simulink library "bcm"  (R2021b)
settings: Solver=VariableStepAuto  StartTime=0.0  StopTime=10.0  RelTol=1e-3
undefined symbols (not defined in the file): ENUM_ANTITHEFT_ALARM, ENUM_ANTITHEFT_ARM, ENUM_ANTITHEFT_DISARM, ENUM_ANTITHEFT_WAIT, ENUM_GEARPOSNTOCAN_P, ENUM_PDKEYRAWLULOCK_INUNLOCK, ENUM_PDKEYRAWPS_INPS, ENUM_POWERSTA_ON, ENUM_POWERSTA_READY, ENUM_POWERSTA_STANDBY, ENUM_PWRSTASW_ON, ENUM_PWRSTASW_READY, ENUM_SYSMODE_DEVELOPING, ENUM_SYSMODE_PRODUCT, ENUM_VEHICLETYPE_D21, ENUM_VEHICLETYPE_D31F25, ENUM_VEHICLETYPE_D31HAWD, ENUM_VEHICLETYPE_D31HRWD, ENUM_VEHICLETYPE_D31L24, FALSE, KBCM_ACCSwcPrsTmr_s, KBCM_ALMBrightnessDark_enum, KBCM_AmbBlue_enum, KBCM_AmbBreathT_ms, KBCM_AmbGreen_enum, KBCM_AmbMidPple_enum, KBCM_AmbRed_enum, KBCM_AmbTempCtrlEN_flg, KBCM_AmbTempT_s, KBCM_AmbWelModeENWait_s, KBCM_Antitheft_enum_ovrdflg, KBCM_Antitheft_enum_ovrdval, KBCM_APMDoorCtrlSta_flg_ovrdflg, KBCM_APMDoorCtrlSta_flg_ovrdval, KBCM_CmdKeepT_s, KBCM_CSWLightRstDebT_s, KBCM_CSWTurnLPRstT_s, KBCM_CycleTimeSet_s, KBCM_DelayTSW_flg, KBCM_DiagDRLOFF_flg, KBCM_DiagFLTC_mA, KBCM_DiagFMHT_s, KBCM_DiagFRTC_mA, KBCM_DiagRLTC_mA, KBCM_DiagRRTC_mA, KBCM_DrAPMRetryTimes_cnt, KBCM_DrOpenWdwOT_s, KBCM_DrOpenWdwReady_s, KBCM_DutyCycleSet_cnt, KBCM_DutyOverride_flg, KBCM_DutyOverride_val, KBCM_ESSOffT_ms, KBCM_ESSOnT_ms, KBCM_FDCDKCReDetectT_K, KBCM_FDCDKCUSSFilterT_K, KBCM_HandleLampKeepT_s, KBCM_IVIRstHoldT_ms, KBCM_IVIRstTriggerT_ms, KBCM_ONDelayT_ms, KBCM_RAPSAbnFlashOFFT_ms ... (+51)
libraries: simulink x402, $bdroot x10, hcu_lib x2
(part 11 of 14)

== system bcm/BCM/BCM/Personal_Setting/PTG/VALUE_TYPE_FlasherSignal ==
  UserNow : Inport
  Loadbar : Inport  Port=2
  iviCMD : Inport  Port=3
  EEP_Set12 : Inport  Port=4
  EEP_Set34 : Inport  Port=5
  EEP_Set57 : Inport  Port=6
  VINP_CANMsgValidIVI2_flg : Inport  Port=7
  NoReqV : Inport  Port=8
  Default : Inport  Port=9
  AND11 : Logic  Operator=OR  AllPortsSameDT=off  OutDataTypeStr=boolean
  Bitwise AND{1..4,11..12} (6 alike) : simulink/Logic and Bit Operations/Bitwise Operator  logicop=AND  UseBitMask=on  BitMask=bin2dec('11111111')  BitMaskRealWorld=Stored Integer
  Bitwise AND10 : simulink/Logic and Bit Operations/Bitwise Operator  logicop=AND  UseBitMask=on  BitMask=bin2dec('00111000')  BitMaskRealWorld=Stored Integer
  Bitwise AND5 : simulink/Logic and Bit Operations/Bitwise Operator  logicop=AND  UseBitMask=on  BitMask=bin2dec('00000111')  BitMaskRealWorld=Stored Integer
  Bitwise AND6 : simulink/Logic and Bit Operations/Bitwise Operator  logicop=AND  UseBitMask=on  BitMask=bin2dec('00111000')  BitMaskRealWorld=Stored Integer
  Bitwise AND7 : simulink/Logic and Bit Operations/Bitwise Operator  logicop=AND  UseBitMask=on  BitMask=bin2dec('00000111')  BitMaskRealWorld=Stored Integer
  Bitwise AND8 : simulink/Logic and Bit Operations/Bitwise Operator  logicop=AND  UseBitMask=on  BitMask=bin2dec('00000111')  BitMaskRealWorld=Stored Integer
  Bitwise AND9 : simulink/Logic and Bit Operations/Bitwise Operator  logicop=AND  UseBitMask=on  BitMask=bin2dec('00111000')  BitMaskRealWorld=Stored Integer
  Bitwise OR1 : simulink/Logic and Bit Operations/Bitwise Operator  logicop=OR  UseBitMask=off  NumInputPorts=2  BitMask=bin2dec('00000000000000000000')  BitMaskRealWorld=Stored Integer
  Bitwise OR2 : simulink/Logic and Bit Operations/Bitwise Operator  logicop=OR  UseBitMask=off  NumInputPorts=2  BitMask=bin2dec('00000000000000000000')  BitMaskRealWorld=Stored Integer
  Bitwise OR3 : simulink/Logic and Bit Operations/Bitwise Operator  logicop=OR  UseBitMask=off  NumInputPorts=2  BitMask=bin2dec('00000000000000000000')  BitMaskRealWorld=Stored Integer
  Compare To Constant5 : simulink/Logic and Bit Operations/Compare To Constant  relop===  const=0  OutDataTypeStr=boolean
  Constant : Constant  OutDataTypeStr=uint8
  Constant1 : Constant  Value=2  OutDataTypeStr=uint8
  Constant2 : Constant  Value=3  OutDataTypeStr=uint8
  Constant3 : Constant  Value=4  OutDataTypeStr=uint8
  Constant4 : Constant  Value=5  OutDataTypeStr=uint8
  Constant5 : Constant  Value=7  OutDataTypeStr=uint8
  Data Type Conversion{,1..14} (15 alike) : DataTypeConversion  OutDataTypeStr=uint8
  Detect Change1 : simulink/Logic and Bit Operations/Detect Change  vinit=0  OutDataTypeStr=boolean
  Detect Change7 : simulink/Logic and Bit Operations/Detect Change  vinit=0  OutDataTypeStr=boolean
  Logical Operator1 : Logic  Inputs=3  AllPortsSameDT=off  OutDataTypeStr=boolean
  Multiport Switch : MultiPortSwitch  Inputs=7  DataPortForDefault=Additional data port  DiagnosticForDefault=None
  NOT : Logic  Operator=NOT  AllPortsSameDT=off  OutDataTypeStr=boolean
  Relational Operator{,1..5} (6 alike) : RelationalOperator  Operator===  OutDataTypeStr=boolean  RndMeth=Simplest
  Relational Operator6 : RelationalOperator  Operator=<  OutDataTypeStr=boolean  RndMeth=Simplest
  Shift Arithmetic1 : ArithShift  BitShiftNumber=3  BitShiftDirection=Left
  Shift Arithmetic2 : ArithShift  BitShiftNumber=3  BitShiftDirection=Left
  Shift Arithmetic3 : ArithShift  BitShiftNumber=3  BitShiftDirection=Right
  Shift Arithmetic4 : ArithShift  BitShiftNumber=3  BitShiftDirection=Right
  Shift Arithmetic5 : ArithShift  BitShiftNumber=3  BitShiftDirection=Right
  Shift Arithmetic6 : ArithShift  BitShiftNumber=3  BitShiftDirection=Left
  Switch{,1..3,5,7..8,12..13} (9 alike) : Switch  Criteria=u2 ~= 0
  Switch{4,6,9..11} (5 alike) : Switch  Criteria=u2 > Threshold
  Unit Delay{1..13} (13 alike) : UnitDelay  SampleTime=-1  HasFrameUpgradeWarning=on
  Setting : Outport
  Set12 : Outport  Port=2
  Set34 : Outport  Port=3
  Set57 : Outport  Port=4
  wires:
  Default/1 -> Multiport Switch/7, Multiport Switch/9
  [Set7] -> Multiport Switch/8
  [Set5] -> Multiport Switch/6
  [Set4] -> Multiport Switch/5
  [Set3] -> Multiport Switch/4
  [Set2] -> Multiport Switch/3
  [Set1] -> Multiport Switch/2
  [Set] -> Switch2/1
  NOT/1 -> Switch1/2
  Switch8/1 -> [Set1], Unit Delay7/1
  Switch10/1 -> [Set5], Unit Delay4/1
  Switch7/1 -> Switch9/1
  Detect Change7/1 -> AND11/2
  Switch3/1 -> Switch4/1
  Relational Operator5/1 -> Unit Delay13/1
  Constant5/1 -> Relational Operator5/2
  [UserNow] -> Relational Operator5/1
  Relational Operator4/1 -> Unit Delay12/1
  Constant4/1 -> Relational Operator4/2
  [UserNow] -> Relational Operator4/1
  Relational Operator3/1 -> Unit Delay11/1
  Constant3/1 -> Relational Operator3/2
  [UserNow] -> Relational Operator3/1
  Relational Operator2/1 -> Unit Delay10/1
  Constant2/1 -> Relational Operator2/2
  [UserNow] -> Relational Operator2/1
  Relational Operator1/1 -> Unit Delay9/1
  Constant1/1 -> Relational Operator1/2
  [UserNow] -> Relational Operator1/1
  [Loadbar] -> Switch8/2
  Switch11/1 -> [Set7], Unit Delay5/1
  [Set] -> Switch7/1
  [Loadbar] -> Switch4/2
  Switch4/1 -> [Set2], Unit Delay2/1
  [UserNow] -> Relational Operator/1
  [Loadbar] -> Switch11/2
  [Loadbar] -> Switch6/2
  Constant/1 -> Relational Operator/2
  [Loadbar] -> Switch10/2
  [Set] -> Switch3/1
  [Set] -> Switch13/1
  Relational Operator/1 -> Unit Delay6/1
  [Set] -> Switch12/1
  [Loadbar] -> Switch9/2
  Switch9/1 -> [Set4], Unit Delay3/1
  [Set] -> Switch5/1
  Switch13/1 -> Switch10/1
  Switch5/1 -> Switch6/1
  Switch12/1 -> Switch11/1
  Switch2/1 -> Switch8/1
  Switch6/1 -> [Set3], Unit Delay8/1
  Relational Operator6/1 -> Logical Operator1/1
  Detect Change1/1 -> Logical Operator1/3
  iviCMD/1 -> Detect Change1/1, Relational Operator6/1, Switch/1
  Multiport Switch/1 -> Switch1/3
  Logical Operator1/1 -> Switch/2
  Switch1/1 -> Switch/3
  AND11/1 -> NOT/1
  Compare To Constant5/1 -> AND11/1
  UserNow/1 -> Multiport Switch/1, [UserNow], Detect Change7/1
  Loadbar/1 -> [Loadbar], Compare To Constant5/1
  Switch/1 -> Unit Delay1/1
  Unit Delay1/1 -> Switch1/1, [Set], Setting/1
  Unit Delay7/1 -> Switch2/3
  Unit Delay2/1 -> Switch3/3
  Unit Delay8/1 -> Switch5/3
  Unit Delay3/1 -> Switch7/3
  Unit Delay4/1 -> Switch13/3
  Unit Delay5/1 -> Switch12/3
  Unit Delay6/1 -> Switch2/2
  Unit Delay9/1 -> Switch3/2
  Unit Delay10/1 -> Switch5/2
  Unit Delay11/1 -> Switch7/2
  Unit Delay12/1 -> Switch13/2
  Unit Delay13/1 -> Switch12/2
  [EEP_Set1] -> Switch8/3
  [EEP_Set2] -> Switch4/3
  [EEP_Set3] -> Switch6/3
  [EEP_Set4] -> Switch9/3
  [EEP_Set5] -> Switch10/3
  [EEP_Set6] -> Switch11/3
  Bitwise AND1/1 -> Bitwise OR1/1
  Shift Arithmetic6/1 -> Bitwise AND2/1
  Data Type Conversion/1 -> Bitwise AND4/1
  Data Type Conversion3/1 -> Bitwise AND1/1
  Shift Arithmetic1/1 -> Bitwise AND11/1
  Data Type Conversion4/1 -> Shift Arithmetic1/1
  Bitwise AND2/1 -> Bitwise OR2/2
  Data Type Conversion1/1 -> Shift Arithmetic6/1
  Bitwise AND11/1 -> Bitwise OR1/2
  Bitwise AND4/1 -> Bitwise OR2/1
  Bitwise OR2/1 -> Set12/1
  Bitwise OR1/1 -> Set34/1
  [Set1] -> Data Type Conversion/1
  [Set2] -> Data Type Conversion1/1
  Bitwise AND9/1 -> Shift Arithmetic4/1
  Bitwise AND5/1 -> Data Type Conversion8/1
  Bitwise AND8/1 -> Data Type Conversion6/1
  Bitwise AND10/1 -> Shift Arithmetic5/1
  Bitwise AND7/1 -> Data Type Conversion10/1
  Shift Arithmetic5/1 -> Data Type Conversion11/1
  Shift Arithmetic4/1 -> Data Type Conversion7/1
  Bitwise AND6/1 -> Shift Arithmetic3/1
  Data Type Conversion6/1 -> [EEP_Set1]
  Data Type Conversion7/1 -> [EEP_Set2]
  Data Type Conversion8/1 -> [EEP_Set3]
  Data Type Conversion9/1 -> [EEP_Set4]
  Data Type Conversion10/1 -> [EEP_Set5]
  Data Type Conversion11/1 -> [EEP_Set6]
  EEP_Set34/1 -> Data Type Conversion13/1
  VINP_CANMsgValidIVI2_flg/1 -> Logical Operator1/2
  [Set3] -> Data Type Conversion3/1
  [Set4] -> Data Type Conversion4/1
  [Set7] -> Data Type Conversion5/1
  [Set5] -> Data Type Conversion2/1
  Bitwise OR3/1 -> Set57/1
  Bitwise AND12/1 -> Bitwise OR3/2
  Data Type Conversion5/1 -> Shift Arithmetic2/1
  Shift Arithmetic2/1 -> Bitwise AND12/1
  Data Type Conversion2/1 -> Bitwise AND3/1
  Bitwise AND3/1 -> Bitwise OR3/1
  EEP_Set57/1 -> Data Type Conversion14/1
  EEP_Set12/1 -> Data Type Conversion12/1
  Data Type Conversion12/1 -> Bitwise AND9/1, Bitwise AND8/1
  Data Type Conversion14/1 -> Bitwise AND10/1, Bitwise AND7/1
  Data Type Conversion13/1 -> Bitwise AND6/1, Bitwise AND5/1
  Shift Arithmetic3/1 -> Data Type Conversion9/1
  NoReqV/1 -> Relational Operator6/2

== system bcm/BCM/BCM/Personal_Setting/PTG/VALUE_TYPE_PTGUserSetMaxHeight ==
  UserNow : Inport
  Loadbar : Inport  Port=2
  VINP_PTGIsSetHeightSta_flg : Inport  Port=3
  VINP_PTGLeftHallPosn_cnt : Inport  Port=4
  EEP_Set1 : Inport  Port=5
  EEP_Set2 : Inport  Port=6
  EEP_Set3 : Inport  Port=7
  EEP_Set4 : Inport  Port=8
  EEP_Set5 : Inport  Port=9
  EEP_Set7 : Inport  Port=10
  NoReqV : Inport  Port=11
  Default : Inport  Port=12
  AND11 : Logic  Operator=OR  AllPortsSameDT=off  OutDataTypeStr=boolean
  Compare To Constant5 : simulink/Logic and Bit Operations/Compare To Constant  relop===  const=0  OutDataTypeStr=boolean
  Constant : Constant  OutDataTypeStr=uint8
  Constant1 : Constant  Value=2  OutDataTypeStr=uint8
  Constant2 : Constant  Value=3  OutDataTypeStr=uint8
  Constant3 : Constant  Value=4  OutDataTypeStr=uint8
  Constant4 : Constant  Value=5  OutDataTypeStr=uint8
  Constant5 : Constant  Value=7  OutDataTypeStr=uint8
  Detect Change7 : simulink/Logic and Bit Operations/Detect Change  vinit=0  OutDataTypeStr=boolean
  Detect Increase : simulink/Logic and Bit Operations/Detect Increase  vinit=0.0  OutDataTypeStr=boolean
  Logical Operator1 : Logic  AllPortsSameDT=off  OutDataTypeStr=boolean
  Multiport Switch : MultiPortSwitch  Inputs=7  DataPortForDefault=Additional data port  DiagnosticForDefault=None
  NOT : Logic  Operator=NOT  AllPortsSameDT=off  OutDataTypeStr=boolean
  Relational Operator{,1..5} (6 alike) : RelationalOperator  Operator===  OutDataTypeStr=boolean  RndMeth=Simplest
  Relational Operator6 : RelationalOperator  Operator=~=  OutDataTypeStr=boolean  RndMeth=Simplest
  Switch{,1..3,5,7..8,12..13} (9 alike) : Switch  Criteria=u2 ~= 0
  Switch{4,6,9..11} (5 alike) : Switch  Criteria=u2 > Threshold
  Unit Delay{1..13} (13 alike) : UnitDelay  SampleTime=-1  HasFrameUpgradeWarning=on
  Setting : Outport
  Set1 : Outport  Port=2
  Set2 : Outport  Port=3
  Set3 : Outport  Port=4
  Set4 : Outport  Port=5
  Set5 : Outport  Port=6
  Set7 : Outport  Port=7
  wires:
  VINP_PTGIsSetHeightSta_flg/1 -> Detect Increase/1
  Default/1 -> Multiport Switch/7, Multiport Switch/9
  [Set7] -> Multiport Switch/8
  [Set5] -> Multiport Switch/6
  [Set4] -> Multiport Switch/5
  [Set3] -> Multiport Switch/4
  [Set2] -> Multiport Switch/3
  [Set1] -> Multiport Switch/2
  [Set] -> Switch2/1
  NOT/1 -> Switch1/2
  Switch8/1 -> [Set1], Unit Delay7/1
  Switch10/1 -> [Set5], Unit Delay4/1
  Switch7/1 -> Switch9/1
  Detect Change7/1 -> AND11/2
  Switch3/1 -> Switch4/1
  Relational Operator5/1 -> Unit Delay13/1
  Constant5/1 -> Relational Operator5/2
  [UserNow] -> Relational Operator5/1
  Relational Operator4/1 -> Unit Delay12/1
  Constant4/1 -> Relational Operator4/2
  [UserNow] -> Relational Operator4/1
  Relational Operator3/1 -> Unit Delay11/1
  Constant3/1 -> Relational Operator3/2
  [UserNow] -> Relational Operator3/1
  Relational Operator2/1 -> Unit Delay10/1
  Constant2/1 -> Relational Operator2/2
  [UserNow] -> Relational Operator2/1
  Relational Operator1/1 -> Unit Delay9/1
  Constant1/1 -> Relational Operator1/2
  [UserNow] -> Relational Operator1/1
  [Loadbar] -> Switch8/2
  EEP_Set3/1 -> Switch6/3
  Switch11/1 -> [Set7], Unit Delay5/1
  EEP_Set4/1 -> Switch9/3
  [Set] -> Switch7/1
  [Loadbar] -> Switch4/2
  Switch4/1 -> [Set2], Unit Delay2/1
  [UserNow] -> Relational Operator/1
  EEP_Set2/1 -> Switch4/3
  EEP_Set5/1 -> Switch10/3
  [Loadbar] -> Switch11/2
  [Loadbar] -> Switch6/2
  Constant/1 -> Relational Operator/2
  [Loadbar] -> Switch10/2
  [Set] -> Switch3/1
  [Set] -> Switch13/1
  Relational Operator/1 -> Unit Delay6/1
  [Set] -> Switch12/1
  [Loadbar] -> Switch9/2
  EEP_Set7/1 -> Switch11/3
  Switch9/1 -> [Set4], Unit Delay3/1
  EEP_Set1/1 -> Switch8/3
  [Set] -> Switch5/1
  Switch13/1 -> Switch10/1
  Switch5/1 -> Switch6/1
  Switch12/1 -> Switch11/1
  Switch2/1 -> Switch8/1
  Switch6/1 -> [Set3], Unit Delay8/1
  NoReqV/1 -> Relational Operator6/1
  Relational Operator6/1 -> Logical Operator1/1
  Detect Increase/1 -> Logical Operator1/2
  VINP_PTGLeftHallPosn_cnt/1 -> Relational Operator6/2, Switch/1
  Multiport Switch/1 -> Switch1/3
  Logical Operator1/1 -> Switch/2
  Switch1/1 -> Switch/3
  [Set1] -> Set1/1
  [Set2] -> Set2/1
  [Set3] -> Set3/1
  [Set4] -> Set4/1
  [Set5] -> Set5/1
  [Set7] -> Set7/1
  AND11/1 -> NOT/1
  Compare To Constant5/1 -> AND11/1
  UserNow/1 -> Multiport Switch/1, [UserNow], Detect Change7/1
  Loadbar/1 -> [Loadbar], Compare To Constant5/1
  Switch/1 -> Unit Delay1/1
  Unit Delay1/1 -> Switch1/1, [Set], Setting/1
  Unit Delay7/1 -> Switch2/3
  Unit Delay2/1 -> Switch3/3
  Unit Delay8/1 -> Switch5/3
  Unit Delay3/1 -> Switch7/3
  Unit Delay4/1 -> Switch13/3
  Unit Delay5/1 -> Switch12/3
  Unit Delay6/1 -> Switch2/2
  Unit Delay9/1 -> Switch3/2
  Unit Delay10/1 -> Switch5/2
  Unit Delay11/1 -> Switch7/2
  Unit Delay12/1 -> Switch13/2
  Unit Delay13/1 -> Switch12/2

== system bcm/BCM/BCM/Personal_Setting/RoomLamp/TOGGLE_TYPE_RoomLampMode ==
  UserNow : Inport
  Loadbar : Inport  Port=2
  iviCMD : Inport  Port=3
  EEP_Set : Inport  Port=4
  Default : Inport  Port=5
  AND : Logic  AllPortsSameDT=off  OutDataTypeStr=boolean
  AND11 : Logic  Operator=OR  AllPortsSameDT=off  OutDataTypeStr=boolean
  Bitwise AND{,1..4} (5 alike) : simulink/Logic and Bit Operations/Bitwise Operator  logicop=AND  UseBitMask=on  BitMask=bin2dec('11111111')  BitMaskRealWorld=Stored Integer
  Bitwise AND10 : simulink/Logic and Bit Operations/Bitwise Operator  logicop=AND  UseBitMask=on  BitMask=bin2dec('00100000')  BitMaskRealWorld=Stored Integer
  Bitwise AND5 : simulink/Logic and Bit Operations/Bitwise Operator  logicop=AND  UseBitMask=on  BitMask=bin2dec('00000001')  BitMaskRealWorld=Stored Integer
  Bitwise AND6 : simulink/Logic and Bit Operations/Bitwise Operator  logicop=AND  UseBitMask=on  BitMask=bin2dec('00000010')  BitMaskRealWorld=Stored Integer
  Bitwise AND7 : simulink/Logic and Bit Operations/Bitwise Operator  logicop=AND  UseBitMask=on  BitMask=bin2dec('00000100')  BitMaskRealWorld=Stored Integer
  Bitwise AND8 : simulink/Logic and Bit Operations/Bitwise Operator  logicop=AND  UseBitMask=on  BitMask=bin2dec('00001000')  BitMaskRealWorld=Stored Integer
  Bitwise AND9 : simulink/Logic and Bit Operations/Bitwise Operator  logicop=AND  UseBitMask=on  BitMask=bin2dec('00010000')  BitMaskRealWorld=Stored Integer
  Bitwise OR2 : simulink/Logic and Bit Operations/Bitwise Operator  logicop=OR  UseBitMask=off  NumInputPorts=6  BitMask=bin2dec('00000000000000000000')  BitMaskRealWorld=Stored Integer
  Compare To Constant5 : simulink/Logic and Bit Operations/Compare To Constant  relop===  const=0  OutDataTypeStr=boolean
  Constant : Constant  OutDataTypeStr=uint8
  Constant1 : Constant  Value=2  OutDataTypeStr=uint8
  Constant2 : Constant  Value=3  OutDataTypeStr=uint8
  Constant3 : Constant  Value=4  OutDataTypeStr=uint8
  Constant4 : Constant  Value=5  OutDataTypeStr=uint8
  Constant5 : Constant  Value=7  OutDataTypeStr=uint8
  Data Type Conversion{,1..5} (6 alike) : DataTypeConversion  OutDataTypeStr=uint8
  Data Type Conversion{6..11} (6 alike) : DataTypeConversion  OutDataTypeStr=boolean
  Detect Change1 : simulink/Logic and Bit Operations/Detect Change  vinit=0  OutDataTypeStr=boolean
  Detect Increase : simulink/Logic and Bit Operations/Detect Increase  vinit=0.0  OutDataTypeStr=boolean
  Multiport Switch : MultiPortSwitch  Inputs=7  DataPortForDefault=Additional data port  DiagnosticForDefault=None
  NOT : Logic  Operator=NOT  IconShape=distinctive  AllPortsSameDT=off  OutDataTypeStr=boolean
  NOT1 : Logic  Operator=NOT  IconShape=distinctive  AllPortsSameDT=off  OutDataTypeStr=boolean
  Relational Operator{,1..5} (6 alike) : RelationalOperator  Operator===  OutDataTypeStr=boolean  RndMeth=Simplest
  Shift Arithmetic1 : ArithShift  BitShiftNumber=4  BitShiftDirection=Left
  Shift Arithmetic10 : ArithShift  BitShiftNumber=5  BitShiftDirection=Right
  Shift Arithmetic2 : ArithShift  BitShiftNumber=5  BitShiftDirection=Left
  Shift Arithmetic3 : ArithShift  BitShiftNumber=1  BitShiftDirection=Right
  Shift Arithmetic4 : ArithShift  BitShiftNumber=2  BitShiftDirection=Right
  Shift Arithmetic5 : ArithShift  BitShiftNumber=3  BitShiftDirection=Right
  Shift Arithmetic6 : ArithShift  BitShiftNumber=1  BitShiftDirection=Left
  Shift Arithmetic7 : ArithShift  BitShiftNumber=2  BitShiftDirection=Left
  Shift Arithmetic8 : ArithShift  BitShiftNumber=3  BitShiftDirection=Left
  Shift Arithmetic9 : ArithShift  BitShiftNumber=4  BitShiftDirection=Right
  Switch{,1..3,5,7,12..13} (8 alike) : Switch  Criteria=u2 ~= 0
  Switch{4,6,8..11} (6 alike) : Switch  Criteria=u2 > Threshold
  Unit Delay{1..4,6..14} (13 alike) : UnitDelay  SampleTime=-1  HasFrameUpgradeWarning=on
  Setting : Outport
  Set : Outport  Port=2
  wires:
  Default/1 -> Multiport Switch/7, Multiport Switch/9
  [Set7] -> Multiport Switch/8
  [Set5] -> Multiport Switch/6
  [Set4] -> Multiport Switch/5
  [Set3] -> Multiport Switch/4
  [Set2] -> Multiport Switch/3
  [Set1] -> Multiport Switch/2
  NOT1/1 -> Switch1/2
  Switch13/1 -> Switch10/1
  Multiport Switch/1 -> Switch1/3
  Loadbar/1 -> [Loadbar], Compare To Constant5/1
  Switch1/1 -> Switch/3
  UserNow/1 -> Multiport Switch/1, [UserNow], Detect Change1/1
  NOT/1 -> Switch/1
  iviCMD/1 -> Detect Increase/1
  [Set] -> Switch13/1
  [Loadbar] -> Switch4/2
  [Set] -> Switch12/1
  [UserNow] -> Relational Operator5/1
  Constant5/1 -> Relational Operator5/2
  [UserNow] -> Relational Operator/1
  [UserNow] -> Relational Operator1/1
  [Loadbar] -> Switch10/2
  Constant2/1 -> Relational Operator2/2
  [Loadbar] -> Switch11/2
  [Set] -> Switch3/1
  Constant/1 -> Relational Operator/2
  [Loadbar] -> Switch9/2
  [UserNow] -> Relational Operator2/1
  [UserNow] -> Relational Operator3/1
  Constant3/1 -> Relational Operator3/2
  [Set] -> Switch2/1
  [UserNow] -> Relational Operator4/1
  Constant1/1 -> Relational Operator1/2
  [Set] -> Switch7/1
  [Loadbar] -> Switch6/2
  [Set] -> Switch5/1
  [Loadbar] -> Switch8/2
  Constant4/1 -> Relational Operator4/2
  Compare To Constant5/1 -> AND11/1
  AND11/1 -> NOT1/1
  Switch/1 -> Unit Delay7/1
  Switch8/1 -> [Set1], Unit Delay6/1
  Switch2/1 -> Switch8/1
  Switch3/1 -> Switch4/1
  Switch4/1 -> [Set2], Unit Delay1/1
  Switch6/1 -> [Set3], Unit Delay11/1
  Switch5/1 -> Switch6/1
  Switch7/1 -> Switch9/1
  Switch9/1 -> [Set4], Unit Delay12/1
  Switch10/1 -> [Set5], Unit Delay13/1
  Switch12/1 -> Switch11/1
  Switch11/1 -> [Set7], Unit Delay14/1
  Unit Delay7/1 -> Setting/1, NOT/1, [Set], Switch1/1
  Relational Operator2/1 -> Unit Delay10/1
  Relational Operator3/1 -> Unit Delay2/1
  Relational Operator4/1 -> Unit Delay3/1
  Relational Operator5/1 -> Unit Delay4/1
  Data Type Conversion2/1 -> Shift Arithmetic7/1
  Data Type Conversion5/1 -> Shift Arithmetic2/1
  [Set4] -> Data Type Conversion3/1
  Shift Arithmetic8/1 -> Bitwise AND/1
  Shift Arithmetic2/1 -> Bitwise AND4/1
  Bitwise AND3/1 -> Bitwise OR2/5
  Bitwise AND1/1 -> Bitwise OR2/3
  Bitwise AND2/1 -> Bitwise OR2/2
  Shift Arithmetic6/1 -> Bitwise AND2/1
  Data Type Conversion4/1 -> Shift Arithmetic1/1
  Shift Arithmetic7/1 -> Bitwise AND1/1
  Shift Arithmetic1/1 -> Bitwise AND3/1
  [Set7] -> Data Type Conversion5/1
  Data Type Conversion/1 -> Bitwise OR2/1
  [Set2] -> Data Type Conversion1/1
  Data Type Conversion3/1 -> Shift Arithmetic8/1
  [Set1] -> Data Type Conversion/1
  [Set5] -> Data Type Conversion4/1
  Bitwise AND/1 -> Bitwise OR2/4
  Data Type Conversion1/1 -> Shift Arithmetic6/1
  Bitwise AND4/1 -> Bitwise OR2/6
  [Set3] -> Data Type Conversion2/1
  Bitwise OR2/1 -> Set/1
  Bitwise AND8/1 -> Shift Arithmetic5/1
  Bitwise AND6/1 -> Shift Arithmetic3/1
  Bitwise AND9/1 -> Shift Arithmetic9/1
  Bitwise AND10/1 -> Shift Arithmetic10/1
  Shift Arithmetic4/1 -> Data Type Conversion8/1
  Shift Arithmetic10/1 -> Data Type Conversion11/1
  Bitwise AND5/1 -> Data Type Conversion6/1
  Shift Arithmetic3/1 -> Data Type Conversion7/1
  Bitwise AND7/1 -> Shift Arithmetic4/1
  Shift Arithmetic9/1 -> Data Type Conversion10/1
  Shift Arithmetic5/1 -> Data Type Conversion9/1
  EEP_Set/1 -> [EEP_Set]
  [EEP_Set] -> Bitwise AND5/1
  [EEP_Set] -> Bitwise AND6/1
  [EEP_Set] -> Bitwise AND7/1
  [EEP_Set] -> Bitwise AND8/1
  [EEP_Set] -> Bitwise AND9/1
  [EEP_Set] -> Bitwise AND10/1
  Data Type Conversion6/1 -> [EEP_Set1]
  Data Type Conversion7/1 -> [EEP_Set2]
  Data Type Conversion8/1 -> [EEP_Set3]
  Data Type Conversion9/1 -> [EEP_Set4]
  Data Type Conversion10/1 -> [EEP_Set5]
  Data Type Conversion11/1 -> [EEP_Set6]
  [EEP_Set1] -> Switch8/3
  [EEP_Set2] -> Switch4/3
  [EEP_Set3] -> Switch6/3
  [EEP_Set4] -> Switch9/3
  [EEP_Set5] -> Switch10/3
  [EEP_Set6] -> Switch11/3
  Relational Operator/1 -> Unit Delay8/1
  Relational Operator1/1 -> Unit Delay9/1
  Unit Delay6/1 -> Switch2/3
  Unit Delay1/1 -> Switch3/3
  Unit Delay8/1 -> Switch2/2
  Unit Delay9/1 -> Switch3/2
  Unit Delay10/1 -> Switch5/2
  Unit Delay11/1 -> Switch5/3
  Unit Delay2/1 -> Switch7/2
  Unit Delay12/1 -> Switch7/3
  Unit Delay3/1 -> Switch13/2
  Unit Delay13/1 -> Switch13/3
  Unit Delay4/1 -> Switch12/2
  Unit Delay14/1 -> Switch12/3
  AND/1 -> Switch/2
  Detect Increase/1 -> AND/2
  [Loadbar] -> AND/1
  Detect Change1/1 -> AND11/2

== system bcm/BCM/BCM/Personal_Setting/SPTG/TOGGLE_TYPE_AmbFunEN ==
  UserNow : Inport
  Loadbar : Inport  Port=2
  iviCMD : Inport  Port=3
  EEP_Set : Inport  Port=4
  Default : Inport  Port=5
  AND : Logic  AllPortsSameDT=off  OutDataTypeStr=boolean
  AND11 : Logic  Operator=OR  AllPortsSameDT=off  OutDataTypeStr=boolean
  Bitwise AND{,1..4} (5 alike) : simulink/Logic and Bit Operations/Bitwise Operator  logicop=AND  UseBitMask=on  BitMask=bin2dec('11111111')  BitMaskRealWorld=Stored Integer
  Bitwise AND10 : simulink/Logic and Bit Operations/Bitwise Operator  logicop=AND  UseBitMask=on  BitMask=bin2dec('00100000')  BitMaskRealWorld=Stored Integer
  Bitwise AND5 : simulink/Logic and Bit Operations/Bitwise Operator  logicop=AND  UseBitMask=on  BitMask=bin2dec('00000001')  BitMaskRealWorld=Stored Integer
  Bitwise AND6 : simulink/Logic and Bit Operations/Bitwise Operator  logicop=AND  UseBitMask=on  BitMask=bin2dec('00000010')  BitMaskRealWorld=Stored Integer
  Bitwise AND7 : simulink/Logic and Bit Operations/Bitwise Operator  logicop=AND  UseBitMask=on  BitMask=bin2dec('00000100')  BitMaskRealWorld=Stored Integer
  Bitwise AND8 : simulink/Logic and Bit Operations/Bitwise Operator  logicop=AND  UseBitMask=on  BitMask=bin2dec('00001000')  BitMaskRealWorld=Stored Integer
  Bitwise AND9 : simulink/Logic and Bit Operations/Bitwise Operator  logicop=AND  UseBitMask=on  BitMask=bin2dec('00010000')  BitMaskRealWorld=Stored Integer
  Bitwise OR2 : simulink/Logic and Bit Operations/Bitwise Operator  logicop=OR  UseBitMask=off  NumInputPorts=6  BitMask=bin2dec('00000000000000000000')  BitMaskRealWorld=Stored Integer
  Compare To Constant5 : simulink/Logic and Bit Operations/Compare To Constant  relop===  const=0  OutDataTypeStr=boolean
  Constant : Constant  OutDataTypeStr=uint8
  Constant1 : Constant  Value=2  OutDataTypeStr=uint8
  Constant2 : Constant  Value=3  OutDataTypeStr=uint8
  Constant3 : Constant  Value=4  OutDataTypeStr=uint8
  Constant4 : Constant  Value=5  OutDataTypeStr=uint8
  Constant5 : Constant  Value=7  OutDataTypeStr=uint8
  Data Type Conversion{,1..5} (6 alike) : DataTypeConversion  OutDataTypeStr=uint8
  Data Type Conversion{6..11} (6 alike) : DataTypeConversion  OutDataTypeStr=boolean
  Detect Change1 : simulink/Logic and Bit Operations/Detect Change  vinit=0  OutDataTypeStr=boolean
  Detect Increase : simulink/Logic and Bit Operations/Detect Increase  vinit=0.0  OutDataTypeStr=boolean
  Multiport Switch : MultiPortSwitch  Inputs=7  DataPortForDefault=Additional data port  DiagnosticForDefault=None
  NOT : Logic  Operator=NOT  IconShape=distinctive  AllPortsSameDT=off  OutDataTypeStr=boolean
  NOT1 : Logic  Operator=NOT  IconShape=distinctive  AllPortsSameDT=off  OutDataTypeStr=boolean
  Relational Operator{,1..5} (6 alike) : RelationalOperator  Operator===  OutDataTypeStr=boolean  RndMeth=Simplest
  Shift Arithmetic1 : ArithShift  BitShiftNumber=4  BitShiftDirection=Left
  Shift Arithmetic10 : ArithShift  BitShiftNumber=5  BitShiftDirection=Right
  Shift Arithmetic2 : ArithShift  BitShiftNumber=5  BitShiftDirection=Left
  Shift Arithmetic3 : ArithShift  BitShiftNumber=1  BitShiftDirection=Right
  Shift Arithmetic4 : ArithShift  BitShiftNumber=2  BitShiftDirection=Right
  Shift Arithmetic5 : ArithShift  BitShiftNumber=3  BitShiftDirection=Right
  Shift Arithmetic6 : ArithShift  BitShiftNumber=1  BitShiftDirection=Left
  Shift Arithmetic7 : ArithShift  BitShiftNumber=2  BitShiftDirection=Left
  Shift Arithmetic8 : ArithShift  BitShiftNumber=3  BitShiftDirection=Left
  Shift Arithmetic9 : ArithShift  BitShiftNumber=4  BitShiftDirection=Right
  Switch{,1..3,5,7,12..13} (8 alike) : Switch  Criteria=u2 ~= 0
  Switch{4,6,8..11} (6 alike) : Switch  Criteria=u2 > Threshold
  Unit Delay{1..4,6..14} (13 alike) : UnitDelay  SampleTime=-1  HasFrameUpgradeWarning=on
  Setting : Outport
  Set : Outport  Port=2
  wires:
  Detect Change1/1 -> AND11/2
  [Loadbar] -> AND/1
  Detect Increase/1 -> AND/2
  AND/1 -> Switch/2
  Unit Delay14/1 -> Switch12/3
  Unit Delay4/1 -> Switch12/2
  Unit Delay13/1 -> Switch13/3
  Unit Delay3/1 -> Switch13/2
  Unit Delay12/1 -> Switch7/3
  Unit Delay2/1 -> Switch7/2
  Unit Delay11/1 -> Switch5/3
  Unit Delay10/1 -> Switch5/2
  Unit Delay9/1 -> Switch3/2
  Unit Delay8/1 -> Switch2/2
  Unit Delay1/1 -> Switch3/3
  Unit Delay6/1 -> Switch2/3
  Relational Operator1/1 -> Unit Delay9/1
  Relational Operator/1 -> Unit Delay8/1
  [EEP_Set6] -> Switch11/3
  [EEP_Set5] -> Switch10/3
  [EEP_Set4] -> Switch9/3
  [EEP_Set3] -> Switch6/3
  [EEP_Set2] -> Switch4/3
  [EEP_Set1] -> Switch8/3
  Data Type Conversion11/1 -> [EEP_Set6]
  Data Type Conversion10/1 -> [EEP_Set5]
  Data Type Conversion9/1 -> [EEP_Set4]
  Data Type Conversion8/1 -> [EEP_Set3]
  Data Type Conversion7/1 -> [EEP_Set2]
  Data Type Conversion6/1 -> [EEP_Set1]
  [EEP_Set] -> Bitwise AND10/1
  [EEP_Set] -> Bitwise AND9/1
  [EEP_Set] -> Bitwise AND8/1
  [EEP_Set] -> Bitwise AND7/1
  [EEP_Set] -> Bitwise AND6/1
  [EEP_Set] -> Bitwise AND5/1
  EEP_Set/1 -> [EEP_Set]
  Shift Arithmetic5/1 -> Data Type Conversion9/1
  Shift Arithmetic9/1 -> Data Type Conversion10/1
  Bitwise AND7/1 -> Shift Arithmetic4/1
  Shift Arithmetic3/1 -> Data Type Conversion7/1
  Bitwise AND5/1 -> Data Type Conversion6/1
  Shift Arithmetic10/1 -> Data Type Conversion11/1
  Shift Arithmetic4/1 -> Data Type Conversion8/1
  Bitwise AND10/1 -> Shift Arithmetic10/1
  Bitwise AND9/1 -> Shift Arithmetic9/1
  Bitwise AND6/1 -> Shift Arithmetic3/1
  Bitwise AND8/1 -> Shift Arithmetic5/1
  Bitwise OR2/1 -> Set/1
  [Set3] -> Data Type Conversion2/1
  Bitwise AND4/1 -> Bitwise OR2/6
  Data Type Conversion1/1 -> Shift Arithmetic6/1
  Bitwise AND/1 -> Bitwise OR2/4
  [Set5] -> Data Type Conversion4/1
  [Set1] -> Data Type Conversion/1
  Data Type Conversion3/1 -> Shift Arithmetic8/1
  [Set2] -> Data Type Conversion1/1
  Data Type Conversion/1 -> Bitwise OR2/1
  [Set7] -> Data Type Conversion5/1
  Shift Arithmetic1/1 -> Bitwise AND3/1
  Shift Arithmetic7/1 -> Bitwise AND1/1
  Data Type Conversion4/1 -> Shift Arithmetic1/1
  Shift Arithmetic6/1 -> Bitwise AND2/1
  Bitwise AND2/1 -> Bitwise OR2/2
  Bitwise AND1/1 -> Bitwise OR2/3
  Bitwise AND3/1 -> Bitwise OR2/5
  Shift Arithmetic2/1 -> Bitwise AND4/1
  Shift Arithmetic8/1 -> Bitwise AND/1
  [Set4] -> Data Type Conversion3/1
  Data Type Conversion5/1 -> Shift Arithmetic2/1
  Data Type Conversion2/1 -> Shift Arithmetic7/1
  Relational Operator5/1 -> Unit Delay4/1
  Relational Operator4/1 -> Unit Delay3/1
  Relational Operator3/1 -> Unit Delay2/1
  Relational Operator2/1 -> Unit Delay10/1
  Unit Delay7/1 -> Switch1/1, [Set], NOT/1, Setting/1
  Switch11/1 -> Unit Delay14/1, [Set7]
  Switch12/1 -> Switch11/1
  Switch10/1 -> Unit Delay13/1, [Set5]
  Switch9/1 -> Unit Delay12/1, [Set4]
  Switch7/1 -> Switch9/1
  Switch5/1 -> Switch6/1
  Switch6/1 -> Unit Delay11/1, [Set3]
  Switch4/1 -> Unit Delay1/1, [Set2]
  Switch3/1 -> Switch4/1
  Switch2/1 -> Switch8/1
  Switch8/1 -> Unit Delay6/1, [Set1]
  Switch/1 -> Unit Delay7/1
  AND11/1 -> NOT1/1
  Compare To Constant5/1 -> AND11/1
  Constant4/1 -> Relational Operator4/2
  [Loadbar] -> Switch8/2
  [Set] -> Switch5/1
  [Loadbar] -> Switch6/2
  [Set] -> Switch7/1
  Constant1/1 -> Relational Operator1/2
  [UserNow] -> Relational Operator4/1
  [Set] -> Switch2/1
  Constant3/1 -> Relational Operator3/2
  [UserNow] -> Relational Operator3/1
  [UserNow] -> Relational Operator2/1
  [Loadbar] -> Switch9/2
  Constant/1 -> Relational Operator/2
  [Set] -> Switch3/1
  [Loadbar] -> Switch11/2
  Constant2/1 -> Relational Operator2/2
  [Loadbar] -> Switch10/2
  [UserNow] -> Relational Operator1/1
  [UserNow] -> Relational Operator/1
  Constant5/1 -> Relational Operator5/2
  [UserNow] -> Relational Operator5/1
  [Set] -> Switch12/1
  [Loadbar] -> Switch4/2
  [Set] -> Switch13/1
  iviCMD/1 -> Detect Increase/1
  NOT/1 -> Switch/1
  UserNow/1 -> Detect Change1/1, [UserNow], Multiport Switch/1
  Switch1/1 -> Switch/3
  Loadbar/1 -> Compare To Constant5/1, [Loadbar]
  Multiport Switch/1 -> Switch1/3
  Switch13/1 -> Switch10/1
  NOT1/1 -> Switch1/2
  [Set1] -> Multiport Switch/2
  [Set2] -> Multiport Switch/3
  [Set3] -> Multiport Switch/4
  [Set4] -> Multiport Switch/5
  [Set5] -> Multiport Switch/6
  [Set7] -> Multiport Switch/8
  Default/1 -> Multiport Switch/9, Multiport Switch/7

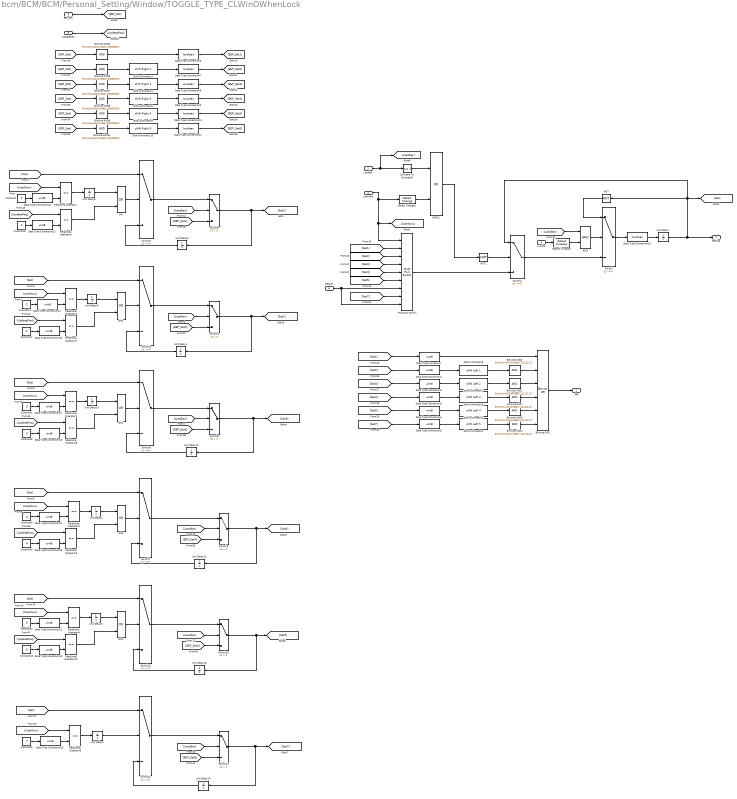
== system bcm/BCM/BCM/Personal_Setting/Window/TOGGLE_TYPE_CLWinOWhenLock ==
  UserNow : Inport
  Loadbar : Inport  Port=2
  UpdateReq : Inport  Port=3
  iviCMD : Inport  Port=4
  EEP_Set : Inport  Port=5
  Default : Inport  Port=6
  AND : Logic  AllPortsSameDT=off  OutDataTypeStr=boolean
  AND11 : Logic  Operator=OR  AllPortsSameDT=off  OutDataTypeStr=boolean
  Bitwise AND{,1..4} (5 alike) : simulink/Logic and Bit Operations/Bitwise Operator  logicop=AND  UseBitMask=on  BitMask=bin2dec('11111111')  BitMaskRealWorld=Stored Integer
  Bitwise AND10 : simulink/Logic and Bit Operations/Bitwise Operator  logicop=AND  UseBitMask=on  BitMask=bin2dec('00100000')  BitMaskRealWorld=Stored Integer
  Bitwise AND5 : simulink/Logic and Bit Operations/Bitwise Operator  logicop=AND  UseBitMask=on  BitMask=bin2dec('00000001')  BitMaskRealWorld=Stored Integer
  Bitwise AND6 : simulink/Logic and Bit Operations/Bitwise Operator  logicop=AND  UseBitMask=on  BitMask=bin2dec('00000010')  BitMaskRealWorld=Stored Integer
  Bitwise AND7 : simulink/Logic and Bit Operations/Bitwise Operator  logicop=AND  UseBitMask=on  BitMask=bin2dec('00000100')  BitMaskRealWorld=Stored Integer
  Bitwise AND8 : simulink/Logic and Bit Operations/Bitwise Operator  logicop=AND  UseBitMask=on  BitMask=bin2dec('00001000')  BitMaskRealWorld=Stored Integer
  Bitwise AND9 : simulink/Logic and Bit Operations/Bitwise Operator  logicop=AND  UseBitMask=on  BitMask=bin2dec('00010000')  BitMaskRealWorld=Stored Integer
  Bitwise OR2 : simulink/Logic and Bit Operations/Bitwise Operator  logicop=OR  UseBitMask=off  NumInputPorts=6  BitMask=bin2dec('00000000000000000000')  BitMaskRealWorld=Stored Integer
  Compare To Constant5 : simulink/Logic and Bit Operations/Compare To Constant  relop===  const=0  OutDataTypeStr=boolean
  Constant : Constant  OutDataTypeStr=uint8
  Constant1 : Constant  Value=2  OutDataTypeStr=uint8
  Constant10 : Constant  Value=5  OutDataTypeStr=uint8
  Constant2 : Constant  Value=3  OutDataTypeStr=uint8
  Constant3 : Constant  Value=4  OutDataTypeStr=uint8
  Constant4 : Constant  Value=5  OutDataTypeStr=uint8
  Constant5 : Constant  Value=7  OutDataTypeStr=uint8
  Constant6 : Constant  OutDataTypeStr=uint8
  Constant7 : Constant  Value=2  OutDataTypeStr=uint8
  Constant8 : Constant  Value=3  OutDataTypeStr=uint8
  Constant9 : Constant  Value=4  OutDataTypeStr=uint8
  Data Type Conversion{,1..5,12..19,21..23} (17 alike) : DataTypeConversion  OutDataTypeStr=uint8
  Data Type Conversion{6..11,20} (7 alike) : DataTypeConversion  OutDataTypeStr=boolean
  Detect Change1 : simulink/Logic and Bit Operations/Detect Change  vinit=0  OutDataTypeStr=boolean
  Detect Increase : simulink/Logic and Bit Operations/Detect Increase  vinit=0.0  OutDataTypeStr=boolean
  Multiport Switch : MultiPortSwitch  Inputs=7  DataPortForDefault=Additional data port  DiagnosticForDefault=None
  NOT : Logic  Operator=NOT  AllPortsSameDT=off  OutDataTypeStr=boolean
  NOT1 : Logic  Operator=NOT  AllPortsSameDT=off  OutDataTypeStr=boolean
  OR{,1..4} (5 alike) : Logic  Operator=OR  AllPortsSameDT=off  OutDataTypeStr=boolean
  Relational Operator{,1..10} (11 alike) : RelationalOperator  Operator===  OutDataTypeStr=boolean  RndMeth=Simplest
  Shift Arithmetic1 : ArithShift  BitShiftNumber=4  BitShiftDirection=Left
  Shift Arithmetic10 : ArithShift  BitShiftNumber=5  BitShiftDirection=Right
  Shift Arithmetic2 : ArithShift  BitShiftNumber=5  BitShiftDirection=Left
  Shift Arithmetic3 : ArithShift  BitShiftNumber=1  BitShiftDirection=Right
  Shift Arithmetic4 : ArithShift  BitShiftNumber=2  BitShiftDirection=Right
  Shift Arithmetic5 : ArithShift  BitShiftNumber=3  BitShiftDirection=Right
  Shift Arithmetic6 : ArithShift  BitShiftNumber=1  BitShiftDirection=Left
  Shift Arithmetic7 : ArithShift  BitShiftNumber=2  BitShiftDirection=Left
  Shift Arithmetic8 : ArithShift  BitShiftNumber=3  BitShiftDirection=Left
  Shift Arithmetic9 : ArithShift  BitShiftNumber=4  BitShiftDirection=Right
  Switch{,1..3,5,7,12..13} (8 alike) : Switch  Criteria=u2 ~= 0
  Switch{4,6,8..11} (6 alike) : Switch  Criteria=u2 > Threshold
  Unit Delay{1..4,6..14} (13 alike) : UnitDelay  SampleTime=-1  HasFrameUpgradeWarning=on
  Setting : Outport
  Set : Outport  Port=2
  wires:
  Default/1 -> Multiport Switch/7, Multiport Switch/9
  [Set7] -> Multiport Switch/8
  [Set5] -> Multiport Switch/6
  [Set4] -> Multiport Switch/5
  [Set3] -> Multiport Switch/4
  [Set2] -> Multiport Switch/3
  [Set1] -> Multiport Switch/2
  NOT1/1 -> Switch1/2
  Switch13/1 -> Switch10/1
  Multiport Switch/1 -> Switch1/3
  Loadbar/1 -> [Loadbar], Compare To Constant5/1
  Switch1/1 -> Switch/3
  UserNow/1 -> Multiport Switch/1, [UserNow], Detect Change1/1
  NOT/1 -> Switch/1
  iviCMD/1 -> Detect Increase/1
  [Set] -> Switch13/1
  [Loadbar] -> Switch4/2
  [Set] -> Switch12/1
  [UserNow] -> Relational Operator5/1
  Constant5/1 -> Data Type Conversion23/1
  [UserNow] -> Relational Operator/1
  [UserNow] -> Relational Operator1/1
  [Loadbar] -> Switch10/2
  Constant2/1 -> Data Type Conversion17/1
  [Loadbar] -> Switch11/2
  [Set] -> Switch3/1
  Constant/1 -> Data Type Conversion12/1
  [Loadbar] -> Switch9/2
  [UserNow] -> Relational Operator2/1
  [UserNow] -> Relational Operator3/1
  Constant3/1 -> Data Type Conversion21/1
  [Set] -> Switch2/1
  [UserNow] -> Relational Operator4/1
  Constant1/1 -> Data Type Conversion14/1
  [Set] -> Switch7/1
  [Loadbar] -> Switch6/2
  [Set] -> Switch5/1
  [Loadbar] -> Switch8/2
  Constant4/1 -> Data Type Conversion22/1
  Compare To Constant5/1 -> AND11/1
  AND11/1 -> NOT1/1
  Switch/1 -> Data Type Conversion20/1
  Switch8/1 -> [Set1], Unit Delay6/1
  Switch2/1 -> Switch8/1
  Switch3/1 -> Switch4/1
  Switch4/1 -> [Set2], Unit Delay1/1
  Switch6/1 -> [Set3], Unit Delay11/1
  Switch5/1 -> Switch6/1
  Switch7/1 -> Switch9/1
  Switch9/1 -> [Set4], Unit Delay12/1
  Switch10/1 -> [Set5], Unit Delay13/1
  Switch12/1 -> Switch11/1
  Switch11/1 -> [Set7], Unit Delay14/1
  Unit Delay7/1 -> Setting/1, NOT/1, [Set], Switch1/1
  Relational Operator2/1 -> Unit Delay10/1
  Relational Operator3/1 -> Unit Delay2/1
  Relational Operator4/1 -> Unit Delay3/1
  Relational Operator5/1 -> Unit Delay4/1
  Data Type Conversion2/1 -> Shift Arithmetic7/1
  Data Type Conversion5/1 -> Shift Arithmetic2/1
  [Set4] -> Data Type Conversion3/1
  Shift Arithmetic8/1 -> Bitwise AND/1
  Shift Arithmetic2/1 -> Bitwise AND4/1
  Bitwise AND3/1 -> Bitwise OR2/5
  Bitwise AND1/1 -> Bitwise OR2/3
  Bitwise AND2/1 -> Bitwise OR2/2
  Shift Arithmetic6/1 -> Bitwise AND2/1
  Data Type Conversion4/1 -> Shift Arithmetic1/1
  Shift Arithmetic7/1 -> Bitwise AND1/1
  Shift Arithmetic1/1 -> Bitwise AND3/1
  [Set7] -> Data Type Conversion5/1
  Data Type Conversion/1 -> Bitwise OR2/1
  [Set2] -> Data Type Conversion1/1
  Data Type Conversion3/1 -> Shift Arithmetic8/1
  [Set1] -> Data Type Conversion/1
  [Set5] -> Data Type Conversion4/1
  Bitwise AND/1 -> Bitwise OR2/4
  Data Type Conversion1/1 -> Shift Arithmetic6/1
  Bitwise AND4/1 -> Bitwise OR2/6
  [Set3] -> Data Type Conversion2/1
  Bitwise OR2/1 -> Set/1
  Bitwise AND8/1 -> Shift Arithmetic5/1
  Bitwise AND6/1 -> Shift Arithmetic3/1
  Bitwise AND9/1 -> Shift Arithmetic9/1
  Bitwise AND10/1 -> Shift Arithmetic10/1
  Shift Arithmetic4/1 -> Data Type Conversion8/1
  Shift Arithmetic10/1 -> Data Type Conversion11/1
  Bitwise AND5/1 -> Data Type Conversion6/1
  Shift Arithmetic3/1 -> Data Type Conversion7/1
  Bitwise AND7/1 -> Shift Arithmetic4/1
  Shift Arithmetic9/1 -> Data Type Conversion10/1
  Shift Arithmetic5/1 -> Data Type Conversion9/1
  EEP_Set/1 -> [EEP_Set]
  [EEP_Set] -> Bitwise AND5/1
  [EEP_Set] -> Bitwise AND6/1
  [EEP_Set] -> Bitwise AND7/1
  [EEP_Set] -> Bitwise AND8/1
  [EEP_Set] -> Bitwise AND9/1
  [EEP_Set] -> Bitwise AND10/1
  Data Type Conversion6/1 -> [EEP_Set1]
  Data Type Conversion7/1 -> [EEP_Set2]
  Data Type Conversion8/1 -> [EEP_Set3]
  Data Type Conversion9/1 -> [EEP_Set4]
  Data Type Conversion10/1 -> [EEP_Set5]
  Data Type Conversion11/1 -> [EEP_Set6]
  [EEP_Set1] -> Switch8/3
  [EEP_Set2] -> Switch4/3
  [EEP_Set3] -> Switch6/3
  [EEP_Set4] -> Switch9/3
  [EEP_Set5] -> Switch10/3
  [EEP_Set6] -> Switch11/3
  Relational Operator/1 -> Unit Delay8/1
  Relational Operator1/1 -> Unit Delay9/1
  Unit Delay6/1 -> Switch2/3
  Unit Delay1/1 -> Switch3/3
  Unit Delay11/1 -> Switch5/3
  Unit Delay12/1 -> Switch7/3
  Unit Delay13/1 -> Switch13/3
  Unit Delay14/1 -> Switch12/3
  AND/1 -> Switch/2
  Detect Increase/1 -> AND/2
  [Loadbar] -> AND/1
  Detect Change1/1 -> AND11/2
  UpdateReq/1 -> [UpdateReq]
  Constant6/1 -> Data Type Conversion13/1
  [UpdateReq] -> Relational Operator6/1
  OR/1 -> Switch2/2
  Unit Delay8/1 -> OR/1
  Relational Operator6/1 -> OR/2
  Relational Operator7/1 -> OR1/2
  [UpdateReq] -> Relational Operator7/1
  OR1/1 -> Switch3/2
  Unit Delay9/1 -> OR1/1
  Data Type Conversion12/1 -> Relational Operator/2
  Data Type Conversion13/1 -> Relational Operator6/2
  Data Type Conversion14/1 -> Relational Operator1/2
  Constant7/1 -> Data Type Conversion15/1
  Data Type Conversion15/1 -> Relational Operator7/2
  Data Type Conversion16/1 -> Relational Operator8/2
  Constant8/1 -> Data Type Conversion16/1
  [UpdateReq] -> Relational Operator8/1
  Relational Operator8/1 -> OR2/2
  OR2/1 -> Switch5/2
  Unit Delay10/1 -> OR2/1
  Data Type Conversion17/1 -> Relational Operator2/2
  Relational Operator9/1 -> OR3/2
  [UpdateReq] -> Relational Operator9/1
  Constant9/1 -> Data Type Conversion18/1
  Data Type Conversion18/1 -> Relational Operator9/2
  OR3/1 -> Switch7/2
  Unit Delay2/1 -> OR3/1
  Data Type Conversion19/1 -> Relational Operator10/2
  Constant10/1 -> Data Type Conversion19/1
  [UpdateReq] -> Relational Operator10/1
  Relational Operator10/1 -> OR4/2
  OR4/1 -> Switch13/2
  Unit Delay3/1 -> OR4/1
  Unit Delay4/1 -> Switch12/2
  Data Type Conversion21/1 -> Relational Operator3/2
  Data Type Conversion22/1 -> Relational Operator4/2
  Data Type Conversion23/1 -> Relational Operator5/2
  Data Type Conversion20/1 -> Unit Delay7/1

== system bcm/BCM/BCM/FlasherSignal/Breath/Duty Cycle/Convert Decrease ==
  Action Port : ActionPort
  Constant2 : Constant  Value=MINUSONE_FLOAT
  ConvertDec : Outport
  wires:
  Constant2/1 -> ConvertDec/1

== system bcm/BCM/BCM/FlasherSignal/Breath/Duty Cycle/Convert Increase ==
  Action Port : ActionPort
  Constant2 : Constant  Value=ONE_FLOAT
  ConvertInc : Outport
  wires:
  Constant2/1 -> ConvertInc/1

== system bcm/BCM/BCM/FlasherSignal/Breath/Duty Cycle/Keep ==
  Keep_Input : Inport
  Action Port : ActionPort
  Keep : Outport
  wires:
  Keep_Input/1 -> Keep/1

== system bcm/BCM/BCM/FlasherSignal/Breath/Duty Cycle/Start ==
  Action Port : ActionPort
  Constant2 : Constant  Value=ONE_FLOAT
  Start : Outport
  wires:
  Constant2/1 -> Start/1

== system bcm/BCM/BCM/FlasherSignal/Breath1/Duty Cycle/Convert Decrease ==
  Action Port : ActionPort
  Constant2 : Constant  Value=MINUSONE_FLOAT
  ConvertDec : Outport
  wires:
  Constant2/1 -> ConvertDec/1

== system bcm/BCM/BCM/FlasherSignal/Breath1/Duty Cycle/Convert Increase ==
  Action Port : ActionPort
  Constant2 : Constant  Value=ONE_FLOAT
  ConvertInc : Outport
  wires:
  Constant2/1 -> ConvertInc/1

== system bcm/BCM/BCM/FlasherSignal/Breath1/Duty Cycle/Keep ==
  Keep_Input : Inport
  Action Port : ActionPort
  Keep : Outport
  wires:
  Keep_Input/1 -> Keep/1

== system bcm/BCM/BCM/FlasherSignal/Breath1/Duty Cycle/Start ==
  Action Port : ActionPort
  Constant2 : Constant  Value=ONE_FLOAT
  Start : Outport
  wires:
  Constant2/1 -> Start/1
